simulink model "Simu_Tiefpass_3O"  (R2015b)
settings: Solver=FixedStepAuto  StartTime=0.0  StopTime=10.0  RelTol=1e-3
libraries: simulink x2
settings Model: Creator=Wolfgang  LastModifiedBy=Wolfgang

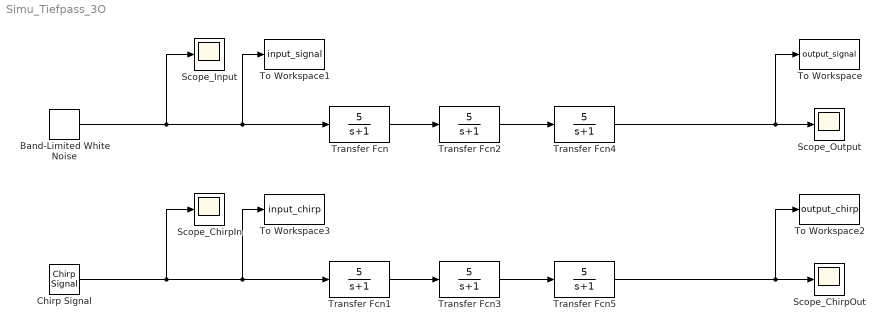
== system Simu_Tiefpass_3O ==
  Band-Limited White Noise : simulink/Sources/Band-Limited White Noise  Cov=[0.01]  Ts=0.1  seed=[23341]
  Chirp Signal : simulink/Sources/Chirp Signal  f1=0.001  T=10  f2=1
  Scope_ChirpIn : Scope
  Scope_ChirpOut : Scope
  Scope_Input : Scope
  Scope_Output : Scope
  To Workspace : ToWorkspace  VariableName=output_signal  SampleTime=-1
  To Workspace1 : ToWorkspace  VariableName=input_signal  SampleTime=-1
  To Workspace2 : ToWorkspace  VariableName=output_chirp  SampleTime=-1
  To Workspace3 : ToWorkspace  VariableName=input_chirp  SampleTime=-1
  Transfer Fcn{,1..5} (6 alike) : TransferFcn  Numerator=[5]  Denominator=[1 1]
  wires:
  Band-Limited White Noise/1 -> Transfer Fcn/1, To Workspace1/1, Scope_Input/1
  Transfer Fcn4/1 -> To Workspace/1, Scope_Output/1
  Chirp Signal/1 -> Transfer Fcn1/1, To Workspace3/1, Scope_ChirpIn/1
  Transfer Fcn5/1 -> To Workspace2/1, Scope_ChirpOut/1
  Transfer Fcn/1 -> Transfer Fcn2/1
  Transfer Fcn1/1 -> Transfer Fcn3/1
  Transfer Fcn2/1 -> Transfer Fcn4/1
  Transfer Fcn3/1 -> Transfer Fcn5/1
